simulink model "lab4"  (R2017b)
settings: Solver=ode45  StartTime=0.0  StopTime=50.0  MaxStep=0.04  RelTol=1e-3
libraries: simulink x1
settings Model: Creator=niquit  LastModifiedBy=niquit

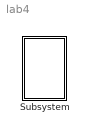
== system lab4 ==
  Subsystem : Subsystem  mask{g=9.81, m1=1, m2=1.4, M=1, R=0.001, r0=2, fi0=90}

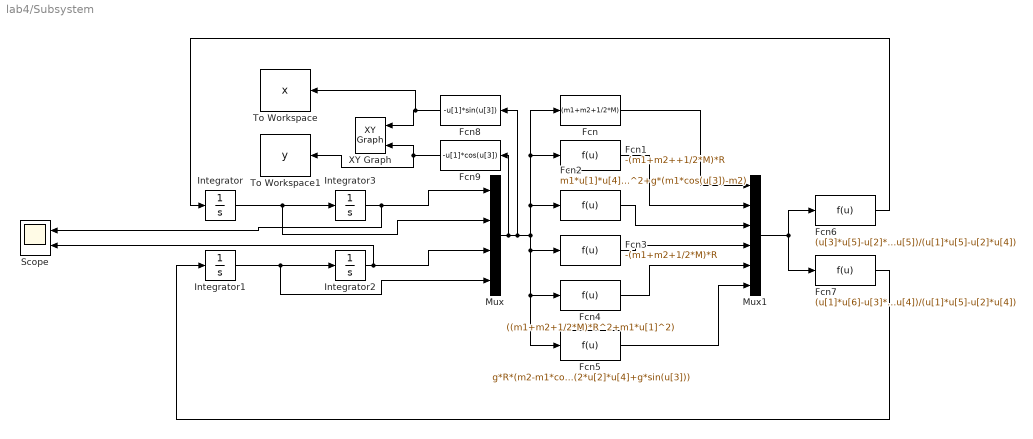
== system lab4/Subsystem ==
  Fcn : Fcn  Expr=(m1+m2+1/2*M)
  Fcn1 : Fcn  Expr=-(m1+m2++1/2*M)*R
  Fcn2 : Fcn  Expr=m1*u[1]*u[4]^2+g*(m1*cos(u[3])-m2)
  Fcn3 : Fcn  Expr=-(m1+m2+1/2*M)*R
  Fcn4 : Fcn  Expr=((m1+m2+1/2*M)*R^2+m1*u[1]^2)
  Fcn5 : Fcn  Expr=g*R*(m2-m1*cos(u[3]))-m1*u[1]*(2*u[2]*u[4]+g*sin(u[3]))
  Fcn6 : Fcn  Expr=(u[3]*u[5]-u[2]*u[5])/(u[1]*u[5]-u[2]*u[4])
  Fcn7 : Fcn  Expr=(u[1]*u[6]-u[3]*u[4])/(u[1]*u[5]-u[2]*u[4])
  Fcn8 : Fcn  Expr=-u[1]*sin(u[3])
  Fcn9 : Fcn  Expr=-u[1]*cos(u[3])
  Integrator : Integrator
  Integrator1 : Integrator
  Integrator2 : Integrator  InitialCondition=fi0*3.14/180
  Integrator3 : Integrator  InitialCondition=r0
  Mux : Mux
  Mux1 : Mux  Inputs=6
  Scope : Scope  NumInputPorts=2
  To Workspace : ToWorkspace  VariableName=x  SampleTime=-1
      settings: Save2DSignal=2-D array (concatenate along first dimension)
  To Workspace1 : ToWorkspace  VariableName=y  SampleTime=-1
      settings: Save2DSignal=2-D array (concatenate along first dimension)
  XY Graph : simulink/Sinks/XY Graph  xmin=-4  xmax=4  ymin=-4  ymax=4  st=-1
  wires:
  Fcn7/1 -> Integrator1/1
  Fcn2/1 -> Mux1/3
  Fcn3/1 -> Mux1/4
  Fcn6/1 -> Integrator/1
  Fcn/1 -> Mux1/1
  Mux/1 -> Fcn9/1, Fcn8/1, Fcn/1, Fcn1/1, Fcn2/1, Fcn5/1, Fcn4/1, Fcn3/1
  Integrator/1 -> Mux/2, Integrator3/1
  Integrator2/1 -> Mux/3, Scope/2
  Fcn1/1 -> Mux1/2
  Integrator3/1 -> Scope/1, Mux/1
  Fcn4/1 -> Mux1/5
  Fcn5/1 -> Mux1/6
  Integrator1/1 -> Mux/4, Integrator2/1
  Mux1/1 -> Fcn6/1, Fcn7/1
  Fcn9/1 -> To Workspace1/1, XY Graph/2
  Fcn8/1 -> To Workspace/1, XY Graph/1
